simulink model "vehicle_dsg"  (R2017a)
settings: Solver=FixedStepDiscrete  StartTime=0.0  StopTime=inf  FixedStep=abs(Ts)  RelTol=1e-3
InitFcn:
  | if ~exist('Ts')
  |     Ts = 1;
  | end
values from neighbouring files (symbols this model uses):
  v = [v1;v2]    [elvio_plot_scatter.m]
undefined symbols (not defined in the file or in its folder): elvio_cycle_wltp_3b, elvio_tag_from
libraries: elvio x17, simulink x3
settings Model: Creator=tstef  LastModifiedBy=tstef

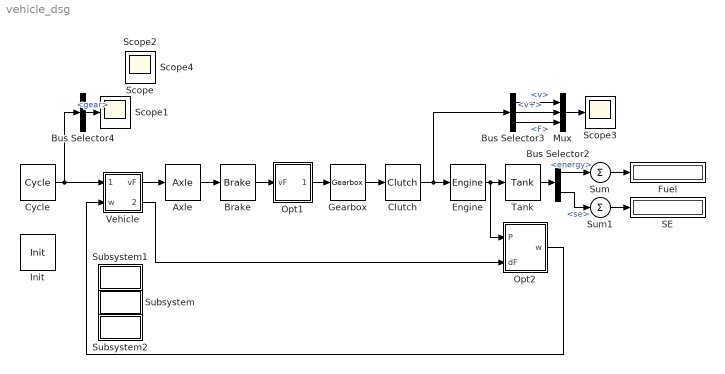
== system vehicle_dsg ==
  Axle : elvio/Drive/Axle  radius=0.3  ratio=4  factor=0.1  FromTag1=Axle1  GotoTag1=MeterV1
  Brake : elvio/Drive/Brake  Tbrake=5000  FromTag1=Brake1  GotoTag1=Axle1
  Bus Selector2 : BusSelector  OutputSignals=energy,se
  Bus Selector3 : BusSelector  OutputSignals=v,v+,F
  Bus Selector4 : BusSelector  OutputSignals=gear
  Clutch : elvio/Drive/Clutch  speed=70  FromTag1=Clutch1  GotoTag1=Gearbox1
  Cycle : elvio/Drive/Cycle  data=elvio_cycle_wltp_3b()  acc=-3
  Engine : elvio/Drive/Engine  Tmax=110  Tmin=0  Tfrict=16  Ploss=800  lossf=0.8  lossnorm=125e3  lossR=0.25  FromTag1=Engine1  GotoTag1=Meter1
  Fuel : Display
  Gearbox : elvio/Drive/Gearbox  gears=[4 2.5 1.8 1.2 0.9 0.9]  factor=0.1  FromTag1=Gearbox1  GotoTag1=Opt21
  Init : elvio/Drive/Init  Ts0=1
  Mux : Mux  Inputs=3
  Opt1 : Subsystem  InitFcn=|  mask(Manual Gearbox){gears=1:5, FromTag1=Opt21, GotoTag1=Brake1}
      | elvio_tag_from([1]);
      | elvio_tag_goto([1]);
      mask prompts: gears "Gears (integer vector):"; FromTag1 "Simulink:blkprm_prompts:FromGotoTag"; GotoTag1 "Simulink:blkprm_prompts:GotoTag"
      mask help: This block is a manual gearbox. It applies to gear chosen by the cycle.
      mask TypeOptions FromTag1: From/GotoTag
      mask TypeOptions GotoTag1: Goto/GotoTag
  Opt2 : Subsystem
  SE : Display
  Scope{,1..4} (5 alike) : Scope
      Scope4 mask Display: disp('1.484e+07')
  Subsystem : Subsystem
      settings: OpenFcn=elvio_plot_scatter(logsout);
      mask Display: disp('Scatter')
  Subsystem1 : Subsystem
      settings: OpenFcn=elvio_plot_energy(logsout);
      mask Display: disp('Energy')
  Subsystem2 : Subsystem
      settings: OpenFcn=elvio_plot_sources(logsout);
      mask Display: disp('Sources')
  Sum : Sum  Inputs=+
  Sum1 : Sum  Inputs=+
  Tank : elvio/Drive/Tank  GotoTag1=Engine1
  Vehicle : Subsystem  InitFcn=elvio_tag_from([1]);  mask(Vehicle Body Model){m=1200, Froll=150, Aeff=0.3, n=[1 5], FromTag1=Vehicle1}
      mask prompts: m "Vehicle Mass (in kg):"; Froll "Tyre Friction (in Nm):"; Aeff "Aero Drag 0.5ρAef (in Ns²/m²):"; n "Number of Simulation (2d):"; FromTag1 "Simulink:blkprm_prompts:FromGotoTag"
      mask help: This block models the inertia and the aerodynamic drag and tyre rolling friction of a vehicle. It turns the cycle into a required tractive effort.
      mask TypeOptions FromTag1: From/GotoTag
  wires:
  Engine/1 -> Opt2/1(P), Tank/1
  Gearbox/1 -> Clutch/1
  Vehicle/1(vF) -> Axle/1
  Bus Selector3/3 -> Mux/3  "<F>"
  Bus Selector3/2 -> Mux/2  "<v+>"
  Mux/1 -> Scope3/1
  Clutch/1 -> Engine/1, Bus Selector3/1
  Bus Selector3/1 -> Mux/1  "<v>"
  Cycle/1 -> Vehicle/1(vreq), Bus Selector4/1
  Bus Selector4/1 -> Scope1/1  "<gear>"
  Axle/1 -> Brake/1
  Opt1/1(vF') -> Gearbox/1
  Opt2/1(w) -> Vehicle/2(w)
  Tank/1 -> Bus Selector2/1
  Brake/1 -> Opt1/1(vF)
  Sum/1 -> Fuel/1
  Bus Selector2/1 -> Sum/1  "<energy>"
  Vehicle/2(dF) -> Opt2/2(dF)
  Sum1/1 -> SE/1
  Bus Selector2/2 -> Sum1/1  "<se>"

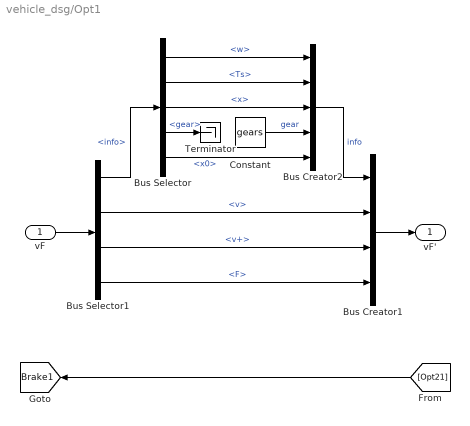
== system vehicle_dsg/Opt1 ==
  vF : Inport
  Bus Creator1 : BusCreator  Inputs=4
  Bus Creator2 : BusCreator  Inputs=5
  Bus Selector : BusSelector  OutputSignals=w,Ts,x,gear,x0
  Bus Selector1 : BusSelector  OutputSignals=info,v,v+,F
  Constant : Constant  Value=gears
  Terminator : Terminator
  vF' : Outport
  tag scope: Brake1=global
  wires:
  [Opt21] -> [Brake1]
  vF/1 -> Bus Selector1/1
  Bus Selector/1 -> Bus Creator2/1  "<w>"
  Bus Selector/2 -> Bus Creator2/2  "<Ts>"
  Bus Selector/3 -> Bus Creator2/3  "<x>"
  Bus Selector/5 -> Bus Creator2/5  "<x0>"
  Bus Creator2/1 -> Bus Creator1/1  "info"
  Bus Selector1/1 -> Bus Selector/1  "<info>"
  Bus Selector1/3 -> Bus Creator1/3  "<v+>"
  Bus Selector1/4 -> Bus Creator1/4  "<F>"
  Bus Selector1/2 -> Bus Creator1/2  "<v>"
  Constant/1 -> Bus Creator2/4  "gear"
  Bus Selector/4 -> Terminator/1  "<gear>"
  Bus Creator1/1 -> vF'/1

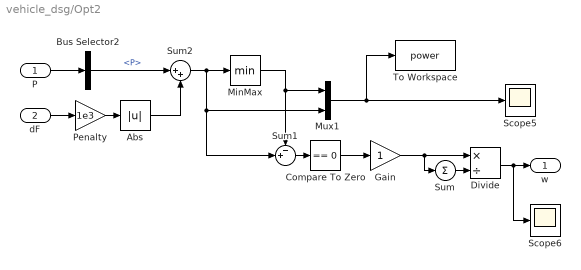
== system vehicle_dsg/Opt2 ==
  P : Inport
  dF : Inport  Port=2
  Abs : Abs
  Bus Selector2 : BusSelector  OutputSignals=P
  Compare To Zero : simulink/Logic and Bit Operations/Compare To Zero  relop===  OutDataTypeStr=boolean
  Divide : Product  Inputs=*/
  Gain : Gain  OutDataTypeStr=double
  MinMax : MinMax
  Mux1 : Mux  Inputs=2
  Penalty : Gain  Gain=1e3
  Scope5 : Scope
  Scope6 : Scope
  Sum : Sum  Inputs=+
  Sum1 : Sum  Inputs=-+|
  Sum2 : Sum  Inputs=|++
  To Workspace : ToWorkspace  VariableName=power  SaveFormat=Timeseries  SampleTime=-1
  w : Outport
  wires:
  P/1 -> Bus Selector2/1
  Mux1/1 -> To Workspace/1, Scope5/1
  Gain/1 -> Sum/1, Divide/1
  Sum1/1 -> Compare To Zero/1
  Sum2/1 -> Mux1/2, Sum1/2, MinMax/1
  Compare To Zero/1 -> Gain/1
  Sum/1 -> Divide/2
  MinMax/1 -> Mux1/1, Sum1/1
  Divide/1 -> w/1, Scope6/1
  dF/1 -> Penalty/1
  Bus Selector2/1 -> Sum2/1  "<P>"
  Penalty/1 -> Abs/1
  Abs/1 -> Sum2/2

== system vehicle_dsg/Subsystem ==

== system vehicle_dsg/Subsystem1 ==

== system vehicle_dsg/Subsystem2 ==

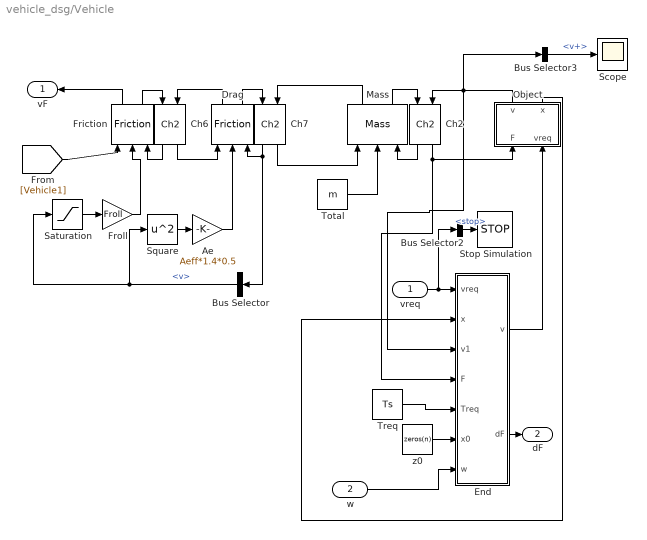
== system vehicle_dsg/Vehicle ==
  vreq : Inport
  w : Inport  Port=2
  Ae : Gain  Gain=Aeff*1.4*0.5
  Bus Selector : BusSelector  OutputSignals=v
  Bus Selector2 : BusSelector  OutputSignals=stop
  Bus Selector3 : BusSelector  OutputSignals=v+
  Ch2 : elvio/Basics/Ch2
  Ch6 : elvio/Basics/Ch2
  Ch7 : elvio/Basics/Ch2
  Drag : elvio/Basics/Friction
  End : Subsystem  AncestorBlock=elvio/Basics/End
  Friction : elvio/Basics/Friction
  Froll : Gain  Gain=Froll
  Mass : elvio/Basics/Mass
  Object : Subsystem  AncestorBlock=elvio/Basics/Object
  Saturation : Saturate  UpperLimit=1  LowerLimit=0  LinearizeAsGain=off  ZeroCross=off
  Scope : Scope
  Square : Math  Operator=square  SaturateOnIntegerOverflow=on
  Stop Simulation : Stop
  Total : Constant  Value=m  VectorParams1D=off
  Treq : Constant  Value=Ts
  z0 : Constant  Value=zeros(n)  VectorParams1D=off
  vF : Outport
  dF : Outport  Port=2
  wires:
  Bus Selector2/1 -> Stop Simulation/1  "<stop>"
  vreq/1 -> End/1(vreq), Bus Selector2/1
  Saturation/1 -> Froll/1
  [Vehicle1] -> Friction/1
  Friction/1 -> vF/1
  Ch2/1 -> Mass/3
  Mass/2 -> Ch2/1
  Ch2/2 -> End/4(F), Object/1(F)
  Object/1(v) -> End/3(v1), Ch2/2, Bus Selector3/1
  z0/1 -> End/6(x0)
  Bus Selector3/1 -> Scope/1  "<v+>"
  Treq/1 -> End/5(Treq)
  End/1(v) -> Object/2(vreq)
  Object/2(x) -> End/2(x)
  Drag/1 -> Ch6/2
  Froll/1 -> Friction/2
  Friction/2 -> Ch6/1
  Ch6/1 -> Friction/3
  Drag/2 -> Ch7/1
  Ch6/2 -> Drag/1
  Ch7/1 -> Bus Selector/1, Drag/3
  Ch7/2 -> Mass/1
  Mass/1 -> Ch7/2
  Bus Selector/1 -> Saturation/1, Square/1  "<v>"
  Total/1 -> Mass/2
  Ae/1 -> Drag/2
  Square/1 -> Ae/1
  w/1 -> End/7(w)
  End/2(dF) -> dF/1

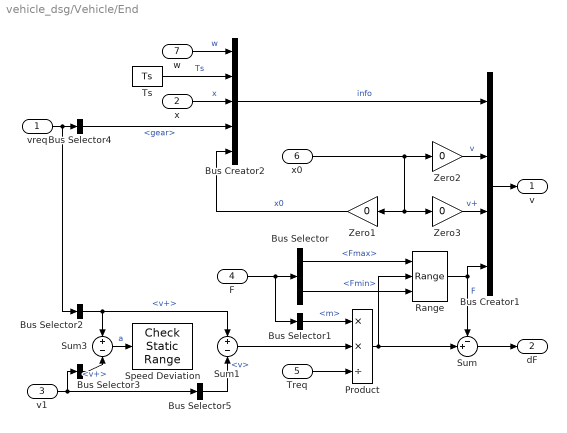
== system vehicle_dsg/Vehicle/End ==
  vreq : Inport
  x : Inport  Port=2  Unit=m/s
  v1 : Inport  Port=3  Unit=m/s
  F : Inport  Port=4  Unit=m/s
  Treq : Inport  Port=5  Unit=m/s
  x0 : Inport  Port=6  Unit=m/s
  w : Inport  Port=7
  Bus Creator1 : BusCreator  Inputs=4
  Bus Creator2 : BusCreator  Inputs=5
  Bus Selector : BusSelector  OutputSignals=Fmax,Fmin
  Bus Selector1 : BusSelector  OutputSignals=m
  Bus Selector2 : BusSelector  OutputSignals=v+
  Bus Selector3 : BusSelector  OutputSignals=v+
  Bus Selector4 : BusSelector  OutputSignals=gear
  Bus Selector5 : BusSelector  OutputSignals=v
  Product : Product  Inputs=**/
  Range : elvio/Utilities/Range
  Speed Deviation : simulink/Model Verification/Check  Static Range  Description=-1 <= u <= 1  max=1  max_included=on  min=-1  min_included=on  enabled=on  stopWhenAssertionFail=off  export=off  icon=graphic
      settings: SourceProductName=Simulink  SourceProductBaseCode=SL
  Sum : Sum  Inputs=-+|
  Sum1 : Sum  Inputs=+-
  Sum3 : Sum  Inputs=+-
  Ts : Constant  Value=Ts
  Zero1 : Gain  Gain=0
  Zero2 : Gain  Gain=0
  Zero3 : Gain  Gain=0
  v : Outport
  dF : Outport  Port=2
  wires:
  Bus Selector2/1 -> Sum1/1, Sum3/1  "<v+>"
  Sum3/1 -> Speed Deviation/1  "a"
  Sum1/1 -> Product/2
  v1/1 -> Bus Selector5/1, Bus Selector3/1
  Bus Selector5/1 -> Sum1/2  "<v>"
  Bus Selector3/1 -> Sum3/2  "<v+>"
  vreq/1 -> Bus Selector4/1, Bus Selector2/1
  Bus Selector4/1 -> Bus Creator2/4  "<gear>"
  Product/1 -> Range/2, Sum/2
  Bus Selector/2 -> Range/3  "<Fmin>"
  Bus Selector/1 -> Range/1  "<Fmax>"
  Bus Selector1/1 -> Product/1  "<m>"
  Ts/1 -> Bus Creator2/2  "Ts"
  Zero1/1 -> Bus Creator2/5  "x0"
  x0/1 -> Zero2/1, Zero1/1, Zero3/1
  Treq/1 -> Product/3
  Zero3/1 -> Bus Creator1/3  "v+"
  Zero2/1 -> Bus Creator1/2  "v"
  Range/1 -> Sum/1, Bus Creator1/4  "F"
  Bus Creator2/1 -> Bus Creator1/1  "info"
  F/1 -> Bus Selector/1, Bus Selector1/1
  Bus Creator1/1 -> v/1
  w/1 -> Bus Creator2/1  "w"
  x/1 -> Bus Creator2/3  "x"
  Sum/1 -> dF/1

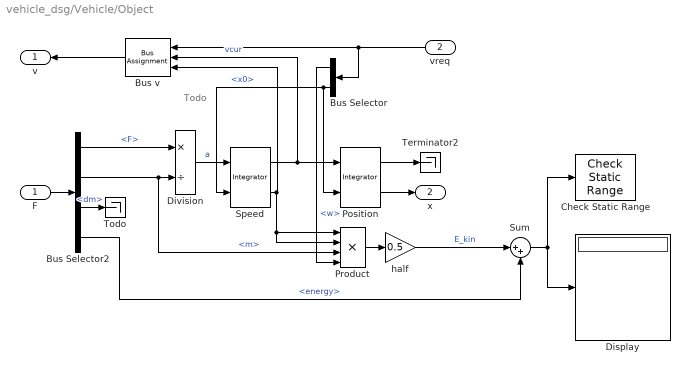
== system vehicle_dsg/Vehicle/Object ==
  note: Todo
  F : Inport
  vreq : Inport  Port=2
  Bus Selector : BusSelector  OutputSignals=info.w,info.x0
  Bus Selector2 : BusSelector  OutputSignals=F,m,dm,energy
  Bus v : BusAssignment  AssignedSignals=v,v+
  Check Static Range : simulink/Model Verification/Check  Static Range  Description=-1e-3 <= u <= 1e-3  max=1e-3  max_included=on  min=-1e-3  min_included=on  enabled=on  stopWhenAssertionFail=off  export=off  icon=graphic
      settings: SourceProductName=Simulink  SourceProductBaseCode=SL
  Display : Display
  Division : Product  Inputs=*/
  Position : elvio/Utilities/Integrator  Ts=Ts
  Product : Product  Inputs=****
  Speed : elvio/Utilities/Integrator  Ts=Ts
  Sum : Sum  Inputs=|++
  Terminator2 : Terminator
  Todo : Terminator
  half : Gain  Gain=0.5
  v : Outport
  x : Outport  Port=2
  wires:
  Sum/1 -> Display/1, Check Static Range/1
  Bus Selector2/4 -> Sum/2  "<energy>"
  Bus Selector/2 -> Speed/2, Position/2  "<x0>"
  Speed/2 -> Bus v/3, Product/1, Product/2
  Position/1 -> Terminator2/1
  Position/2 -> x/1
  Bus Selector/1 -> Product/4  "<w>"
  Bus v/1 -> v/1
  Bus Selector2/3 -> Todo/1  "<dm>"
  half/1 -> Sum/1  "E_kin"
  F/1 -> Bus Selector2/1
  Bus Selector2/1 -> Division/1  "<F>"
  Product/1 -> half/1
  Division/1 -> Speed/1  "a"
  Speed/1 -> Bus v/2, Position/1  "vcur"
  Bus Selector2/2 -> Division/2, Product/3  "<m>"
  vreq/1 -> Bus v/1, Bus Selector/1
